simulink model "AVIC_model"  (R2015b)
settings: Solver=ode45  StartTime=0.0  StopTime=simtime  RelTol=1e-3
values from neighbouring files (symbols this model uses):
  A = 1    [simulation.m]
  a1 = 1    [simulation.m]
  a2 = 3    [simulation.m]
  a3 = 3    [simulation.m]
  Amp1 = Ampl/1000000    (= 134.217728)    [simulation.m]
  b1 = 1    [simulation.m]
  B2 = 8    [simulation.m]
  C = 32    [simulation.m]
  c1 = 1    [simulation.m]
  c2 = 1    [simulation.m]
  c3 = 1    [simulation.m]
  finrad = 2*pi/(N)*f0*clk    [simulation.m]
  FSC = 2^27    (= 134217728)    [simulation.m]
  SAT = 127    [simulation.m]
  Ts = 1/clk    (= 1.62760416667e-07)    [simulation.m]
libraries: simulink x298
(part 2 of 5)

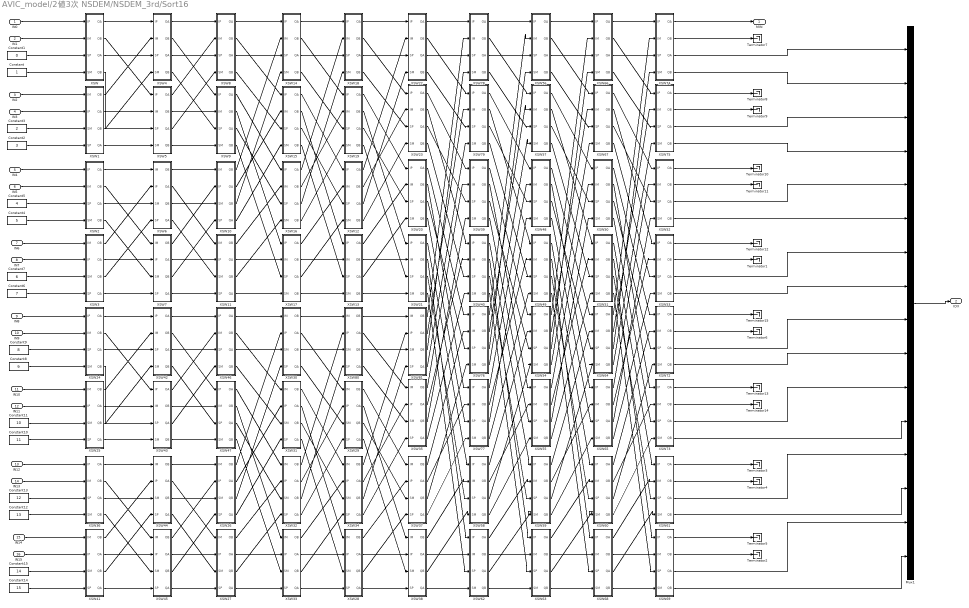
== system AVIC_model/2値3次 NSDEM/NSDEM_3rd/Sort16 ==
  IN0 : Inport
  IN1 : Inport  Port=2
  IN2 : Inport  Port=3
  IN3 : Inport  Port=4
  IN4 : Inport  Port=5
  IN5 : Inport  Port=6
  IN6 : Inport  Port=7
  IN7 : Inport  Port=8
  IN8 : Inport  Port=9
  IN9 : Inport  Port=10
  IN10 : Inport  Port=11
  IN11 : Inport  Port=12
  IN12 : Inport  Port=13
  IN13 : Inport  Port=14
  IN14 : Inport  Port=15
  IN15 : Inport  Port=16
  Constant : Constant
  Constant1 : Constant  Value=0
  Constant10 : Constant  Value=11
  Constant11 : Constant  Value=10
  Constant12 : Constant  Value=13
  Constant13 : Constant  Value=12
  Constant14 : Constant  Value=15
  Constant15 : Constant  Value=14
  Constant2 : Constant  Value=3
  Constant3 : Constant  Value=2
  Constant4 : Constant  Value=5
  Constant5 : Constant  Value=4
  Constant6 : Constant  Value=7
  Constant7 : Constant  Value=6
  Constant8 : Constant  Value=9
  Constant9 : Constant  Value=8
  Mux1 : Mux  Inputs=16
  Terminator{1..15} (15 alike) : Terminator
  XSW : Subsystem
  XSW1 : Subsystem
  XSW10 : Subsystem
  XSW11 : Subsystem
  XSW12 : Subsystem
  XSW13 : Subsystem
  XSW14 : Subsystem
  XSW15 : Subsystem
  XSW16 : Subsystem
  XSW17 : Subsystem
  XSW18 : Subsystem
  XSW19 : Subsystem
  XSW2 : Subsystem
  XSW20 : Subsystem
  XSW21 : Subsystem
  XSW22 : Subsystem
  XSW23 : Subsystem
  XSW24 : Subsystem
  XSW25 : Subsystem
  XSW26 : Subsystem
  XSW27 : Subsystem
  XSW28 : Subsystem
  XSW29 : Subsystem
  XSW3 : Subsystem
  XSW30 : Subsystem
  XSW31 : Subsystem
  XSW32 : Subsystem
  XSW33 : Subsystem
  XSW34 : Subsystem
  XSW35 : Subsystem
  XSW36 : Subsystem
  XSW37 : Subsystem
  XSW38 : Subsystem
  XSW39 : Subsystem
  XSW4 : Subsystem
  XSW40 : Subsystem
  XSW41 : Subsystem
  XSW42 : Subsystem
  XSW43 : Subsystem
  XSW44 : Subsystem
  XSW45 : Subsystem
  XSW46 : Subsystem
  XSW47 : Subsystem
  XSW48 : Subsystem
  XSW49 : Subsystem
  XSW5 : Subsystem
  XSW50 : Subsystem
  XSW51 : Subsystem
  XSW52 : Subsystem
  XSW53 : Subsystem
  XSW54 : Subsystem
  XSW55 : Subsystem
  XSW56 : Subsystem
  XSW57 : Subsystem
  XSW58 : Subsystem
  XSW59 : Subsystem
  XSW6 : Subsystem
  XSW60 : Subsystem
  XSW61 : Subsystem
  XSW62 : Subsystem
  XSW63 : Subsystem
  XSW64 : Subsystem
  XSW65 : Subsystem
  XSW66 : Subsystem
  XSW67 : Subsystem
  XSW68 : Subsystem
  XSW69 : Subsystem
  XSW7 : Subsystem
  XSW72 : Subsystem
  XSW73 : Subsystem
  XSW74 : Subsystem
  XSW75 : Subsystem
  XSW76 : Subsystem
  XSW77 : Subsystem
  XSW78 : Subsystem
  XSW79 : Subsystem
  XSW8 : Subsystem
  XSW80 : Subsystem
  XSW81 : Subsystem
  XSW9 : Subsystem
  MIN : Outport
  IDX : Outport  Port=2
  wires:
  XSW/1(OA) -> XSW4/1(IP)
  XSW/2(OB) -> XSW5/1(IP)
  XSW/3(QA) -> XSW4/3(SP)
  XSW/4(QB) -> XSW5/3(SP)
  XSW1/4(QA) -> XSW5/4(SM)
  XSW1/3(QB) -> XSW4/4(SM)
  XSW1/2(OA) -> XSW5/2(IM)
  XSW1/1(OB) -> XSW4/2(IM)
  XSW2/1(OA) -> XSW6/1(IM)
  XSW2/2(OB) -> XSW7/1(IM)
  XSW2/3(QA) -> XSW6/3(SM)
  XSW2/4(QB) -> XSW7/3(SM)
  XSW3/4(QA) -> XSW7/4(SP)
  XSW3/2(OA) -> XSW7/2(IP)
  XSW3/3(QB) -> XSW6/4(SP)
  XSW3/1(OB) -> XSW6/2(IP)
  XSW4/1(OA) -> XSW8/1(IP)
  XSW4/3(QA) -> XSW8/3(SP)
  XSW4/2(OB) -> XSW9/1(IP)
  XSW4/4(QB) -> XSW9/3(SP)
  XSW5/4(QB) -> XSW9/4(SM)
  XSW5/2(OB) -> XSW9/2(IM)
  XSW5/3(QA) -> XSW8/4(SM)
  XSW5/1(OA) -> XSW8/2(IM)
  XSW6/1(OB) -> XSW10/1(IM)
  XSW6/3(QB) -> XSW10/3(SM)
  XSW6/2(OA) -> XSW11/1(IM)
  XSW6/4(QA) -> XSW11/3(SM)
  XSW7/4(QA) -> XSW11/4(SP)
  XSW7/2(OA) -> XSW11/2(IP)
  XSW7/3(QB) -> XSW10/4(SP)
  XSW7/1(OB) -> XSW10/2(IP)
  XSW8/1(OA) -> XSW14/1(IP)
  XSW8/2(OB) -> XSW15/1(IP)
  XSW9/1(OA) -> XSW16/1(IP)
  XSW9/2(OB) -> XSW17/1(IP)
  XSW11/4(QA) -> XSW17/4(SM)
  XSW11/2(OA) -> XSW17/2(IM)
  XSW11/3(QB) -> XSW16/4(SM)
  XSW11/1(OB) -> XSW16/2(IM)
  XSW8/3(QA) -> XSW14/3(SP)
  XSW8/4(QB) -> XSW15/3(SP)
  XSW9/3(QA) -> XSW16/3(SP)
  XSW9/4(QB) -> XSW17/3(SP)
  XSW10/4(QA) -> XSW15/4(SM)
  XSW10/2(OA) -> XSW15/2(IM)
  XSW10/3(QB) -> XSW14/4(SM)
  XSW10/1(OB) -> XSW14/2(IM)
  XSW14/1(OA) -> XSW18/1(IP)
  XSW14/3(QA) -> XSW18/3(SP)
  XSW14/2(OB) -> XSW19/1(IP)
  XSW14/4(QB) -> XSW19/3(SP)
  XSW15/1(OA) -> XSW12/1(IP)
  XSW15/3(QA) -> XSW12/3(SP)
  XSW15/2(OB) -> XSW13/1(IP)
  XSW15/4(QB) -> XSW13/3(SP)
  XSW17/4(QB) -> XSW13/4(SM)
  XSW17/2(OB) -> XSW13/2(IM)
  XSW17/3(QA) -> XSW12/4(SM)
  XSW17/1(OA) -> XSW12/2(IM)
  XSW16/4(QB) -> XSW19/4(SM)
  XSW16/2(OB) -> XSW19/2(IM)
  XSW16/3(QA) -> XSW18/4(SM)
  XSW16/1(OA) -> XSW18/2(IM)
  XSW18/1(OA) -> XSW22/1(IP)
  XSW18/3(QA) -> XSW22/3(SP)
  XSW18/2(OB) -> XSW23/1(IP)
  XSW18/4(QB) -> XSW23/3(SP)
  XSW19/1(OA) -> XSW20/1(IP)
  XSW19/3(QA) -> XSW20/3(SP)
  XSW19/2(OB) -> XSW21/1(IP)
  XSW19/4(QB) -> XSW21/3(SP)
  XSW13/4(QB) -> XSW21/4(SM)
  XSW13/2(OB) -> XSW21/2(IM)
  XSW13/3(QA) -> XSW20/4(SM)
  XSW13/1(OA) -> XSW20/2(IM)
  XSW12/4(QB) -> XSW23/4(SM)
  XSW12/2(OB) -> XSW23/2(IM)
  XSW12/3(QA) -> XSW22/4(SM)
  XSW12/1(OA) -> XSW22/2(IM)
  XSW24/1(OA) -> XSW42/1(IP)
  XSW24/2(OB) -> XSW43/1(IP)
  XSW24/3(QA) -> XSW42/3(SP)
  XSW24/4(QB) -> XSW43/3(SP)
  XSW25/4(QA) -> XSW43/4(SM)
  XSW25/3(QB) -> XSW42/4(SM)
  XSW25/2(OA) -> XSW43/2(IM)
  XSW25/1(OB) -> XSW42/2(IM)
  XSW36/1(OA) -> XSW44/1(IM)
  XSW36/2(OB) -> XSW45/1(IM)
  XSW36/3(QA) -> XSW44/3(SM)
  XSW36/4(QB) -> XSW45/3(SM)
  XSW41/4(QA) -> XSW45/4(SP)
  XSW41/2(OA) -> XSW45/2(IP)
  XSW41/3(QB) -> XSW44/4(SP)
  XSW41/1(OB) -> XSW44/2(IP)
  XSW42/1(OA) -> XSW46/1(IP)
  XSW42/3(QA) -> XSW46/3(SP)
  XSW42/2(OB) -> XSW47/1(IP)
  XSW42/4(QB) -> XSW47/3(SP)
  XSW43/4(QB) -> XSW47/4(SM)
  XSW43/2(OB) -> XSW47/2(IM)
  XSW43/3(QA) -> XSW46/4(SM)
  XSW43/1(OA) -> XSW46/2(IM)
  XSW44/1(OB) -> XSW26/1(IM)
  XSW44/3(QB) -> XSW26/3(SM)
  XSW44/2(OA) -> XSW27/1(IM)
  XSW44/4(QA) -> XSW27/3(SM)
  XSW45/4(QA) -> XSW27/4(SP)
  XSW45/2(OA) -> XSW27/2(IP)
  XSW45/3(QB) -> XSW26/4(SP)
  XSW45/1(OB) -> XSW26/2(IP)
  XSW46/1(OA) -> XSW30/1(IM)
  XSW46/2(OB) -> XSW31/1(IM)
  XSW47/1(OA) -> XSW32/1(IM)
  XSW47/2(OB) -> XSW33/1(IM)
  XSW27/4(QA) -> XSW33/4(SP)
  XSW27/2(OA) -> XSW33/2(IP)
  XSW27/3(QB) -> XSW32/4(SP)
  XSW27/1(OB) -> XSW32/2(IP)
  XSW46/3(QA) -> XSW30/3(SM)
  XSW46/4(QB) -> XSW31/3(SM)
  XSW47/3(QA) -> XSW32/3(SM)
  XSW47/4(QB) -> XSW33/3(SM)
  XSW26/4(QA) -> XSW31/4(SP)
  XSW26/2(OA) -> XSW31/2(IP)
  XSW26/3(QB) -> XSW30/4(SP)
  XSW26/1(OB) -> XSW30/2(IP)
  XSW30/1(OB) -> XSW80/1(IM)
  XSW30/3(QB) -> XSW80/3(SM)
  XSW30/2(OA) -> XSW29/1(IM)
  XSW30/4(QA) -> XSW29/3(SM)
  XSW31/1(OB) -> XSW34/1(IM)
  XSW31/3(QB) -> XSW34/3(SM)
  XSW31/2(OA) -> XSW28/1(IM)
  XSW31/4(QA) -> XSW28/3(SM)
  XSW33/4(QA) -> XSW28/4(SP)
  XSW33/2(OA) -> XSW28/2(IP)
  XSW33/3(QB) -> XSW34/4(SP)
  XSW33/1(OB) -> XSW34/2(IP)
  XSW32/4(QA) -> XSW29/4(SP)
  XSW32/2(OA) -> XSW29/2(IP)
  XSW32/3(QB) -> XSW80/4(SP)
  XSW32/1(OB) -> XSW80/2(IP)
  XSW80/1(OB) -> XSW81/1(IM)
  XSW80/3(QB) -> XSW81/3(SM)
  XSW80/2(OA) -> XSW35/1(IM)
  XSW80/4(QA) -> XSW35/3(SM)
  XSW29/1(OB) -> XSW37/1(IM)
  XSW29/3(QB) -> XSW37/3(SM)
  XSW29/2(OA) -> XSW38/1(IM)
  XSW29/4(QA) -> XSW38/3(SM)
  XSW28/4(QA) -> XSW38/4(SP)
  XSW28/2(OA) -> XSW38/2(IP)
  XSW28/3(QB) -> XSW37/4(SP)
  XSW28/1(OB) -> XSW37/2(IP)
  XSW34/4(QA) -> XSW35/4(SP)
  XSW34/2(OA) -> XSW35/2(IP)
  XSW34/3(QB) -> XSW81/4(SP)
  XSW34/1(OB) -> XSW81/2(IP)
  XSW22/1(OA) -> XSW78/1(IP)
  XSW22/2(OB) -> XSW79/1(IP)
  XSW23/1(OA) -> XSW39/1(IP)
  XSW23/2(OB) -> XSW40/1(IP)
  XSW20/1(OA) -> XSW76/1(IP)
  XSW20/2(OB) -> XSW77/1(IP)
  XSW21/1(OA) -> XSW58/1(IP)
  XSW21/2(OB) -> XSW62/1(IP)
  XSW81/1(OB) -> XSW78/2(IM)
  XSW81/2(OA) -> XSW79/2(IM)
  XSW35/1(OB) -> XSW39/2(IM)
  XSW35/2(OA) -> XSW40/2(IM)
  XSW37/1(OB) -> XSW76/2(IM)
  XSW37/2(OA) -> XSW77/2(IM)
  XSW38/1(OB) -> XSW58/2(IM)
  XSW38/2(OA) -> XSW62/2(IM)
  XSW22/3(QA) -> XSW78/3(SP)
  XSW22/4(QB) -> XSW79/3(SP)
  XSW23/3(QA) -> XSW39/3(SP)
  XSW23/4(QB) -> XSW40/3(SP)
  XSW20/3(QA) -> XSW76/3(SP)
  XSW20/4(QB) -> XSW77/3(SP)
  XSW21/3(QA) -> XSW58/3(SP)
  XSW21/4(QB) -> XSW62/3(SP)
  XSW81/3(QB) -> XSW78/4(SM)
  XSW81/4(QA) -> XSW79/4(SM)
  XSW35/3(QB) -> XSW39/4(SM)
  XSW35/4(QA) -> XSW40/4(SM)
  XSW37/3(QB) -> XSW76/4(SM)
  XSW37/4(QA) -> XSW77/4(SM)
  XSW38/3(QB) -> XSW58/4(SM)
  XSW38/4(QA) -> XSW62/4(SM)
  XSW78/1(OA) -> XSW56/1(IP)
  XSW78/2(OB) -> XSW57/1(IP)
  XSW79/1(OA) -> XSW48/1(IP)
  XSW79/2(OB) -> XSW49/1(IP)
  XSW39/1(OA) -> XSW54/1(IP)
  XSW39/2(OB) -> XSW55/1(IP)
  XSW40/1(OA) -> XSW59/1(IP)
  XSW40/2(OB) -> XSW63/1(IP)
  XSW76/1(OA) -> XSW56/2(IM)
  XSW76/2(OB) -> XSW57/2(IM)
  XSW77/1(OA) -> XSW48/2(IM)
  XSW77/2(OB) -> XSW49/2(IM)
  XSW58/1(OA) -> XSW54/2(IM)
  XSW58/2(OB) -> XSW55/2(IM)
  XSW62/1(OA) -> XSW59/2(IM)
  XSW62/2(OB) -> XSW63/2(IM)
  XSW78/3(QA) -> XSW56/3(SP)
  XSW78/4(QB) -> XSW57/3(SP)
  XSW79/3(QA) -> XSW48/3(SP)
  XSW79/4(QB) -> XSW49/3(SP)
  XSW39/3(QA) -> XSW54/3(SP)
  XSW39/4(QB) -> XSW55/3(SP)
  XSW40/3(QA) -> XSW59/3(SP)
  XSW40/4(QB) -> XSW63/3(SP)
  XSW76/3(QA) -> XSW56/4(SM)
  XSW76/4(QB) -> XSW57/4(SM)
  XSW77/3(QA) -> XSW48/4(SM)
  XSW77/4(QB) -> XSW49/4(SM)
  XSW58/3(QA) -> XSW54/4(SM)
  XSW58/4(QB) -> XSW55/4(SM)
  XSW62/3(QA) -> XSW59/4(SM)
  XSW62/4(QB) -> XSW63/4(SM)
  XSW56/1(OA) -> XSW66/1(IP)
  XSW56/2(OB) -> XSW67/1(IP)
  XSW57/1(OA) -> XSW50/1(IP)
  XSW57/2(OB) -> XSW51/1(IP)
  XSW48/1(OA) -> XSW64/1(IP)
  XSW48/2(OB) -> XSW65/1(IP)
  XSW49/1(OA) -> XSW60/1(IP)
  XSW49/2(OB) -> XSW68/1(IP)
  XSW54/1(OA) -> XSW66/2(IM)
  XSW54/2(OB) -> XSW67/2(IM)
  XSW55/1(OA) -> XSW50/2(IM)
  XSW55/2(OB) -> XSW51/2(IM)
  XSW59/1(OA) -> XSW64/2(IM)
  XSW59/2(OB) -> XSW65/2(IM)
  XSW63/1(OA) -> XSW60/2(IM)
  XSW63/2(OB) -> XSW68/2(IM)
  XSW56/3(QA) -> XSW66/3(SP)
  XSW56/4(QB) -> XSW67/3(SP)
  XSW57/3(QA) -> XSW50/3(SP)
  XSW57/4(QB) -> XSW51/3(SP)
  XSW48/3(QA) -> XSW64/3(SP)
  XSW48/4(QB) -> XSW65/3(SP)
  XSW49/3(QA) -> XSW60/3(SP)
  XSW49/4(QB) -> XSW68/3(SP)
  XSW54/3(QA) -> XSW66/4(SM)
  XSW54/4(QB) -> XSW67/4(SM)
  XSW55/3(QA) -> XSW50/4(SM)
  XSW55/4(QB) -> XSW51/4(SM)
  XSW59/3(QA) -> XSW64/4(SM)
  XSW59/4(QB) -> XSW65/4(SM)
  XSW63/3(QA) -> XSW60/4(SM)
  XSW63/4(QB) -> XSW68/4(SM)
  XSW66/1(OA) -> XSW74/1(IP)
  XSW66/2(OB) -> XSW75/1(IP)
  XSW67/1(OA) -> XSW52/1(IP)
  XSW67/2(OB) -> XSW53/1(IP)
  XSW50/1(OA) -> XSW72/1(IP)
  XSW50/2(OB) -> XSW73/1(IP)
  XSW51/1(OA) -> XSW61/1(IP)
  XSW51/2(OB) -> XSW69/1(IP)
  XSW64/1(OA) -> XSW74/2(IM)
  XSW64/2(OB) -> XSW75/2(IM)
  XSW65/1(OA) -> XSW52/2(IM)
  XSW65/2(OB) -> XSW53/2(IM)
  XSW60/1(OA) -> XSW72/2(IM)
  XSW60/2(OB) -> XSW73/2(IM)
  XSW68/1(OA) -> XSW61/2(IM)
  XSW68/2(OB) -> XSW69/2(IM)
  XSW66/3(QA) -> XSW74/3(SP)
  XSW66/4(QB) -> XSW75/3(SP)
  XSW67/3(QA) -> XSW52/3(SP)
  XSW67/4(QB) -> XSW53/3(SP)
  XSW50/3(QA) -> XSW72/3(SP)
  XSW50/4(QB) -> XSW73/3(SP)
  XSW51/3(QA) -> XSW61/3(SP)
  XSW51/4(QB) -> XSW69/3(SP)
  XSW64/3(QA) -> XSW74/4(SM)
  XSW64/4(QB) -> XSW75/4(SM)
  XSW65/3(QA) -> XSW52/4(SM)
  XSW65/4(QB) -> XSW53/4(SM)
  XSW60/3(QA) -> XSW72/4(SM)
  XSW60/4(QB) -> XSW73/4(SM)
  XSW68/3(QA) -> XSW61/4(SM)
  XSW68/4(QB) -> XSW69/4(SM)
  XSW74/1(OA) -> MIN/1
  XSW74/2(OB) -> Terminator7/1
  XSW75/1(OA) -> Terminator8/1
  XSW75/2(OB) -> Terminator9/1
  XSW52/1(OA) -> Terminator10/1
  XSW52/2(OB) -> Terminator11/1
  XSW53/1(OA) -> Terminator12/1
  XSW53/2(OB) -> Terminator1/1
  XSW72/1(OA) -> Terminator15/1
  XSW72/2(OB) -> Terminator6/1
  XSW73/1(OA) -> Terminator13/1
  XSW73/2(OB) -> Terminator14/1
  XSW61/1(OA) -> Terminator3/1
  XSW61/2(OB) -> Terminator4/1
  XSW69/1(OA) -> Terminator5/1
  XSW69/2(OB) -> Terminator2/1
  IN0/1 -> XSW/1(IP)
  IN1/1 -> XSW/2(IM)
  Constant1/1 -> XSW/3(SP)
  Constant/1 -> XSW/4(SM)
  IN2/1 -> XSW1/1(IM)
  IN3/1 -> XSW1/2(IP)
  Constant3/1 -> XSW1/3(SM)
  Constant2/1 -> XSW1/4(SP)
  IN4/1 -> XSW2/1(IP)
  IN5/1 -> XSW2/2(IM)
  Constant5/1 -> XSW2/3(SP)
  Constant4/1 -> XSW2/4(SM)
  IN6/1 -> XSW3/1(IM)
  IN7/1 -> XSW3/2(IP)
  Constant7/1 -> XSW3/3(SM)
  Constant6/1 -> XSW3/4(SP)
  IN8/1 -> XSW24/1(IP)
  IN9/1 -> XSW24/2(IM)
  Constant9/1 -> XSW24/3(SP)
  Constant8/1 -> XSW24/4(SM)
  IN10/1 -> XSW25/1(IM)
  IN11/1 -> XSW25/2(IP)
  Constant11/1 -> XSW25/3(SM)
  Constant10/1 -> XSW25/4(SP)
  IN12/1 -> XSW36/1(IP)
  IN13/1 -> XSW36/2(IM)
  Constant13/1 -> XSW36/3(SP)
  Constant12/1 -> XSW36/4(SM)
  IN14/1 -> XSW41/1(IM)
  IN15/1 -> XSW41/2(IP)
  Constant15/1 -> XSW41/3(SM)
  Constant14/1 -> XSW41/4(SP)
  XSW53/4(QB) -> Mux1/8
  XSW74/3(QA) -> Mux1/1
  XSW74/4(QB) -> Mux1/2
  XSW75/3(QA) -> Mux1/3
  XSW75/4(QB) -> Mux1/4
  XSW52/3(QA) -> Mux1/5
  XSW52/4(QB) -> Mux1/6
  XSW53/3(QA) -> Mux1/7
  XSW72/3(QA) -> Mux1/9
  XSW72/4(QB) -> Mux1/10
  XSW73/3(QA) -> Mux1/11
  XSW73/4(QB) -> Mux1/12
  XSW61/3(QA) -> Mux1/13
  XSW61/4(QB) -> Mux1/14
  XSW69/3(QA) -> Mux1/15
  XSW69/4(QB) -> Mux1/16
  Mux1/1 -> IDX/1

== system AVIC_model/ESB/Subsystem4/Subsystem ==
  In1 : Inport
  Combinatorial Logic{,2,4..5} (4 alike) : CombinatorialLogic  TruthTable=[0 0 0 0 0 0 0 0;0 0 0 0 0 0 0 0]
  Combinatorial Logic1 : CombinatorialLogic  TruthTable=[0 0 0 0 0 0 0 0;0 0 0 0 0 0 0 1]
  Combinatorial Logic3 : CombinatorialLogic  TruthTable=[0 0 0 0 0 0 0 0;0 0 0 0 0 0 0 1]
  Compare To Constnt : simulink/Logic and Bit Operations/Compare To Constant  relop===  const=0  OutDataTypeStr=boolean  ZeroCross=off
  Compare To Constnt1 : simulink/Logic and Bit Operations/Compare To Constant  relop===  const=1  OutDataTypeStr=boolean  ZeroCross=off
  Compare To Constnt2 : simulink/Logic and Bit Operations/Compare To Constant  relop===  const=2  OutDataTypeStr=boolean  ZeroCross=off
  Logical Operator : Logic  Operator=OR  Inputs=3  AllPortsSameDT=off  OutDataTypeStr=boolean
  Logical Operator1 : Logic  Operator=OR  Inputs=3  AllPortsSameDT=off  OutDataTypeStr=boolean
  "P1 " : Outport
  "N1 " : Outport  Port=2
  wires:
  Logical Operator/1 -> "P1 "/1
  In1/1 -> Compare To Constnt/1, Compare To Constnt1/1, Compare To Constnt2/1
  Combinatorial Logic/1 -> Logical Operator/1
  Combinatorial Logic2/1 -> Logical Operator/2
  Combinatorial Logic1/1 -> Logical Operator/3
  Logical Operator1/1 -> "N1 "/1
  Compare To Constnt/1 -> Combinatorial Logic3/1, Combinatorial Logic/1
  Compare To Constnt1/1 -> Combinatorial Logic4/1, Combinatorial Logic2/1
  Compare To Constnt2/1 -> Combinatorial Logic5/1, Combinatorial Logic1/1
  Combinatorial Logic3/1 -> Logical Operator1/1
  Combinatorial Logic4/1 -> Logical Operator1/2
  Combinatorial Logic5/1 -> Logical Operator1/3

== system AVIC_model/ESB/Subsystem4/Subsystem1 ==
  In1 : Inport
  Combinatorial Logic{,2,4..5} (4 alike) : CombinatorialLogic  TruthTable=[0 0 0 0 0 0 0 0;0 0 0 0 0 0 0 0]
  Combinatorial Logic1 : CombinatorialLogic  TruthTable=[0 0 0 0 0 0 0 0;0 0 0 0 0 0 1 0]
  Combinatorial Logic3 : CombinatorialLogic  TruthTable=[0 0 0 0 0 0 0 0;0 0 0 0 0 0 1 0]
  Compare To Constnt : simulink/Logic and Bit Operations/Compare To Constant  relop===  const=0  OutDataTypeStr=boolean  ZeroCross=off
  Compare To Constnt1 : simulink/Logic and Bit Operations/Compare To Constant  relop===  const=1  OutDataTypeStr=boolean  ZeroCross=off
  Compare To Constnt2 : simulink/Logic and Bit Operations/Compare To Constant  relop===  const=2  OutDataTypeStr=boolean  ZeroCross=off
  Logical Operator : Logic  Operator=OR  Inputs=3  AllPortsSameDT=off  OutDataTypeStr=boolean
  Logical Operator1 : Logic  Operator=OR  Inputs=3  AllPortsSameDT=off  OutDataTypeStr=boolean
  "P1 " : Outport
  "N1 " : Outport  Port=2
  wires:
  Logical Operator/1 -> "P1 "/1
  In1/1 -> Compare To Constnt/1, Compare To Constnt1/1, Compare To Constnt2/1
  Combinatorial Logic/1 -> Logical Operator/1
  Combinatorial Logic2/1 -> Logical Operator/2
  Combinatorial Logic1/1 -> Logical Operator/3
  Logical Operator1/1 -> "N1 "/1
  Compare To Constnt/1 -> Combinatorial Logic3/1, Combinatorial Logic/1
  Compare To Constnt1/1 -> Combinatorial Logic4/1, Combinatorial Logic2/1
  Compare To Constnt2/1 -> Combinatorial Logic5/1, Combinatorial Logic1/1
  Combinatorial Logic3/1 -> Logical Operator1/1
  Combinatorial Logic4/1 -> Logical Operator1/2
  Combinatorial Logic5/1 -> Logical Operator1/3

== system AVIC_model/ESB/Subsystem4/Subsystem2 ==
  In1 : Inport
  Combinatorial Logic{,2,4..5} (4 alike) : CombinatorialLogic  TruthTable=[0 0 0 0 0 0 0 0;0 0 0 0 0 0 0 0]
  Combinatorial Logic1 : CombinatorialLogic  TruthTable=[0 0 0 0 0 0 0 0;0 0 0 0 0 1 0 0]
  Combinatorial Logic3 : CombinatorialLogic  TruthTable=[0 0 0 0 0 0 0 0;0 0 0 0 0 1 0 0]
  Compare To Constnt : simulink/Logic and Bit Operations/Compare To Constant  relop===  const=0  OutDataTypeStr=boolean  ZeroCross=off
  Compare To Constnt1 : simulink/Logic and Bit Operations/Compare To Constant  relop===  const=1  OutDataTypeStr=boolean  ZeroCross=off
  Compare To Constnt2 : simulink/Logic and Bit Operations/Compare To Constant  relop===  const=2  OutDataTypeStr=boolean  ZeroCross=off
  Logical Operator : Logic  Operator=OR  Inputs=3  AllPortsSameDT=off  OutDataTypeStr=boolean
  Logical Operator1 : Logic  Operator=OR  Inputs=3  AllPortsSameDT=off  OutDataTypeStr=boolean
  "P1 " : Outport
  "N1 " : Outport  Port=2
  wires:
  Logical Operator/1 -> "P1 "/1
  In1/1 -> Compare To Constnt/1, Compare To Constnt1/1, Compare To Constnt2/1
  Combinatorial Logic/1 -> Logical Operator/1
  Combinatorial Logic2/1 -> Logical Operator/2
  Combinatorial Logic1/1 -> Logical Operator/3
  Logical Operator1/1 -> "N1 "/1
  Compare To Constnt/1 -> Combinatorial Logic3/1, Combinatorial Logic/1
  Compare To Constnt1/1 -> Combinatorial Logic4/1, Combinatorial Logic2/1
  Compare To Constnt2/1 -> Combinatorial Logic5/1, Combinatorial Logic1/1
  Combinatorial Logic3/1 -> Logical Operator1/1
  Combinatorial Logic4/1 -> Logical Operator1/2
  Combinatorial Logic5/1 -> Logical Operator1/3

== system AVIC_model/ESB/Subsystem4/Subsystem3 ==
  In1 : Inport
  Combinatorial Logic{,2,4..5} (4 alike) : CombinatorialLogic  TruthTable=[0 0 0 0 0 0 0 0;0 0 0 0 0 0 0 0]
  Combinatorial Logic1 : CombinatorialLogic  TruthTable=[0 0 0 0 0 0 0 0;0 0 0 0 1 0 0 0]
  Combinatorial Logic3 : CombinatorialLogic  TruthTable=[0 0 0 0 0 0 0 0;0 0 0 0 1 0 0 0]
  Compare To Constnt : simulink/Logic and Bit Operations/Compare To Constant  relop===  const=0  OutDataTypeStr=boolean  ZeroCross=off
  Compare To Constnt1 : simulink/Logic and Bit Operations/Compare To Constant  relop===  const=1  OutDataTypeStr=boolean  ZeroCross=off
  Compare To Constnt2 : simulink/Logic and Bit Operations/Compare To Constant  relop===  const=2  OutDataTypeStr=boolean  ZeroCross=off
  Logical Operator : Logic  Operator=OR  Inputs=3  AllPortsSameDT=off  OutDataTypeStr=boolean
  Logical Operator1 : Logic  Operator=OR  Inputs=3  AllPortsSameDT=off  OutDataTypeStr=boolean
  "P1 " : Outport
  "N1 " : Outport  Port=2
  wires:
  Logical Operator/1 -> "P1 "/1
  In1/1 -> Compare To Constnt/1, Compare To Constnt1/1, Compare To Constnt2/1
  Combinatorial Logic/1 -> Logical Operator/1
  Combinatorial Logic2/1 -> Logical Operator/2
  Combinatorial Logic1/1 -> Logical Operator/3
  Logical Operator1/1 -> "N1 "/1
  Compare To Constnt/1 -> Combinatorial Logic3/1, Combinatorial Logic/1
  Compare To Constnt1/1 -> Combinatorial Logic4/1, Combinatorial Logic2/1
  Compare To Constnt2/1 -> Combinatorial Logic5/1, Combinatorial Logic1/1
  Combinatorial Logic3/1 -> Logical Operator1/1
  Combinatorial Logic4/1 -> Logical Operator1/2
  Combinatorial Logic5/1 -> Logical Operator1/3

== system AVIC_model/ESB/Subsystem4/Subsystem4 ==
  In1 : Inport
  Combinatorial Logic{,2,4..5} (4 alike) : CombinatorialLogic  TruthTable=[0 0 0 0 0 0 0 0;0 0 0 0 0 0 0 0]
  Combinatorial Logic1 : CombinatorialLogic  TruthTable=[0 0 0 0 0 0 0 0;0 0 0 1 0 0 0 0]
  Combinatorial Logic3 : CombinatorialLogic  TruthTable=[0 0 0 0 0 0 0 0;0 0 0 1 0 0 0 0]
  Compare To Constnt : simulink/Logic and Bit Operations/Compare To Constant  relop===  const=0  OutDataTypeStr=boolean  ZeroCross=off
  Compare To Constnt1 : simulink/Logic and Bit Operations/Compare To Constant  relop===  const=1  OutDataTypeStr=boolean  ZeroCross=off
  Compare To Constnt2 : simulink/Logic and Bit Operations/Compare To Constant  relop===  const=2  OutDataTypeStr=boolean  ZeroCross=off
  Logical Operator : Logic  Operator=OR  Inputs=3  AllPortsSameDT=off  OutDataTypeStr=boolean
  Logical Operator1 : Logic  Operator=OR  Inputs=3  AllPortsSameDT=off  OutDataTypeStr=boolean
  "P1 " : Outport
  "N1 " : Outport  Port=2
  wires:
  Logical Operator/1 -> "P1 "/1
  In1/1 -> Compare To Constnt/1, Compare To Constnt1/1, Compare To Constnt2/1
  Combinatorial Logic/1 -> Logical Operator/1
  Combinatorial Logic2/1 -> Logical Operator/2
  Combinatorial Logic1/1 -> Logical Operator/3
  Logical Operator1/1 -> "N1 "/1
  Compare To Constnt/1 -> Combinatorial Logic3/1, Combinatorial Logic/1
  Compare To Constnt1/1 -> Combinatorial Logic4/1, Combinatorial Logic2/1
  Compare To Constnt2/1 -> Combinatorial Logic5/1, Combinatorial Logic1/1
  Combinatorial Logic3/1 -> Logical Operator1/1
  Combinatorial Logic4/1 -> Logical Operator1/2
  Combinatorial Logic5/1 -> Logical Operator1/3

== system AVIC_model/ESB/Subsystem4/Subsystem5 ==
  In1 : Inport
  Combinatorial Logic{,2,4..5} (4 alike) : CombinatorialLogic  TruthTable=[0 0 0 0 0 0 0 0;0 0 0 0 0 0 0 0]
  Combinatorial Logic1 : CombinatorialLogic  TruthTable=[0 0 0 0 0 0 0 0;0 0 1 0 0 0 0 0]
  Combinatorial Logic3 : CombinatorialLogic  TruthTable=[0 0 0 0 0 0 0 0;0 0 1 0 0 0 0 0]
  Compare To Constnt : simulink/Logic and Bit Operations/Compare To Constant  relop===  const=0  OutDataTypeStr=boolean  ZeroCross=off
  Compare To Constnt1 : simulink/Logic and Bit Operations/Compare To Constant  relop===  const=1  OutDataTypeStr=boolean  ZeroCross=off
  Compare To Constnt2 : simulink/Logic and Bit Operations/Compare To Constant  relop===  const=2  OutDataTypeStr=boolean  ZeroCross=off
  Logical Operator : Logic  Operator=OR  Inputs=3  AllPortsSameDT=off  OutDataTypeStr=boolean
  Logical Operator1 : Logic  Operator=OR  Inputs=3  AllPortsSameDT=off  OutDataTypeStr=boolean
  "P1 " : Outport
  "N1 " : Outport  Port=2
  wires:
  Logical Operator/1 -> "P1 "/1
  In1/1 -> Compare To Constnt/1, Compare To Constnt1/1, Compare To Constnt2/1
  Combinatorial Logic/1 -> Logical Operator/1
  Combinatorial Logic2/1 -> Logical Operator/2
  Combinatorial Logic1/1 -> Logical Operator/3
  Logical Operator1/1 -> "N1 "/1
  Compare To Constnt/1 -> Combinatorial Logic3/1, Combinatorial Logic/1
  Compare To Constnt1/1 -> Combinatorial Logic4/1, Combinatorial Logic2/1
  Compare To Constnt2/1 -> Combinatorial Logic5/1, Combinatorial Logic1/1
  Combinatorial Logic3/1 -> Logical Operator1/1
  Combinatorial Logic4/1 -> Logical Operator1/2
  Combinatorial Logic5/1 -> Logical Operator1/3

== system AVIC_model/ESB/Subsystem4/Subsystem6 ==
  In1 : Inport
  Combinatorial Logic{,2,4..5} (4 alike) : CombinatorialLogic  TruthTable=[0 0 0 0 0 0 0 0;0 0 0 0 0 0 0 0]
  Combinatorial Logic1 : CombinatorialLogic  TruthTable=[0 0 0 0 0 0 0 0;0 1 0 0 0 0 0 0]
  Combinatorial Logic3 : CombinatorialLogic  TruthTable=[0 0 0 0 0 0 0 0;0 1 0 0 0 0 0 0]
  Compare To Constnt : simulink/Logic and Bit Operations/Compare To Constant  relop===  const=0  OutDataTypeStr=boolean  ZeroCross=off
  Compare To Constnt1 : simulink/Logic and Bit Operations/Compare To Constant  relop===  const=1  OutDataTypeStr=boolean  ZeroCross=off
  Compare To Constnt2 : simulink/Logic and Bit Operations/Compare To Constant  relop===  const=2  OutDataTypeStr=boolean  ZeroCross=off
  Logical Operator : Logic  Operator=OR  Inputs=3  AllPortsSameDT=off  OutDataTypeStr=boolean
  Logical Operator1 : Logic  Operator=OR  Inputs=3  AllPortsSameDT=off  OutDataTypeStr=boolean
  "P1 " : Outport
  "N1 " : Outport  Port=2
  wires:
  Logical Operator/1 -> "P1 "/1
  In1/1 -> Compare To Constnt/1, Compare To Constnt1/1, Compare To Constnt2/1
  Combinatorial Logic/1 -> Logical Operator/1
  Combinatorial Logic2/1 -> Logical Operator/2
  Combinatorial Logic1/1 -> Logical Operator/3
  Logical Operator1/1 -> "N1 "/1
  Compare To Constnt/1 -> Combinatorial Logic3/1, Combinatorial Logic/1
  Compare To Constnt1/1 -> Combinatorial Logic4/1, Combinatorial Logic2/1
  Compare To Constnt2/1 -> Combinatorial Logic5/1, Combinatorial Logic1/1
  Combinatorial Logic3/1 -> Logical Operator1/1
  Combinatorial Logic4/1 -> Logical Operator1/2
  Combinatorial Logic5/1 -> Logical Operator1/3

== system AVIC_model/ESB/Subsystem4/Subsystem7 ==
  In1 : Inport
  Combinatorial Logic{,2,4..5} (4 alike) : CombinatorialLogic  TruthTable=[0 0 0 0 0 0 0 0;0 0 0 0 0 0 0 0]
  Combinatorial Logic1 : CombinatorialLogic  TruthTable=[0 0 0 0 0 0 0 0;1 0 0 0 0 0 0 0]
  Combinatorial Logic3 : CombinatorialLogic  TruthTable=[0 0 0 0 0 0 0 0;1 0 0 0 0 0 0 0]
  Compare To Constnt : simulink/Logic and Bit Operations/Compare To Constant  relop===  const=0  OutDataTypeStr=boolean  ZeroCross=off
  Compare To Constnt1 : simulink/Logic and Bit Operations/Compare To Constant  relop===  const=1  OutDataTypeStr=boolean  ZeroCross=off
  Compare To Constnt2 : simulink/Logic and Bit Operations/Compare To Constant  relop===  const=2  OutDataTypeStr=boolean  ZeroCross=off
  Logical Operator : Logic  Operator=OR  Inputs=3  AllPortsSameDT=off  OutDataTypeStr=boolean
  Logical Operator1 : Logic  Operator=OR  Inputs=3  AllPortsSameDT=off  OutDataTypeStr=boolean
  "P1 " : Outport
  "N1 " : Outport  Port=2
  wires:
  Logical Operator/1 -> "P1 "/1
  In1/1 -> Compare To Constnt/1, Compare To Constnt1/1, Compare To Constnt2/1
  Combinatorial Logic/1 -> Logical Operator/1
  Combinatorial Logic2/1 -> Logical Operator/2
  Combinatorial Logic1/1 -> Logical Operator/3
  Logical Operator1/1 -> "N1 "/1
  Compare To Constnt/1 -> Combinatorial Logic3/1, Combinatorial Logic/1
  Compare To Constnt1/1 -> Combinatorial Logic4/1, Combinatorial Logic2/1
  Compare To Constnt2/1 -> Combinatorial Logic5/1, Combinatorial Logic1/1
  Combinatorial Logic3/1 -> Logical Operator1/1
  Combinatorial Logic4/1 -> Logical Operator1/2
  Combinatorial Logic5/1 -> Logical Operator1/3

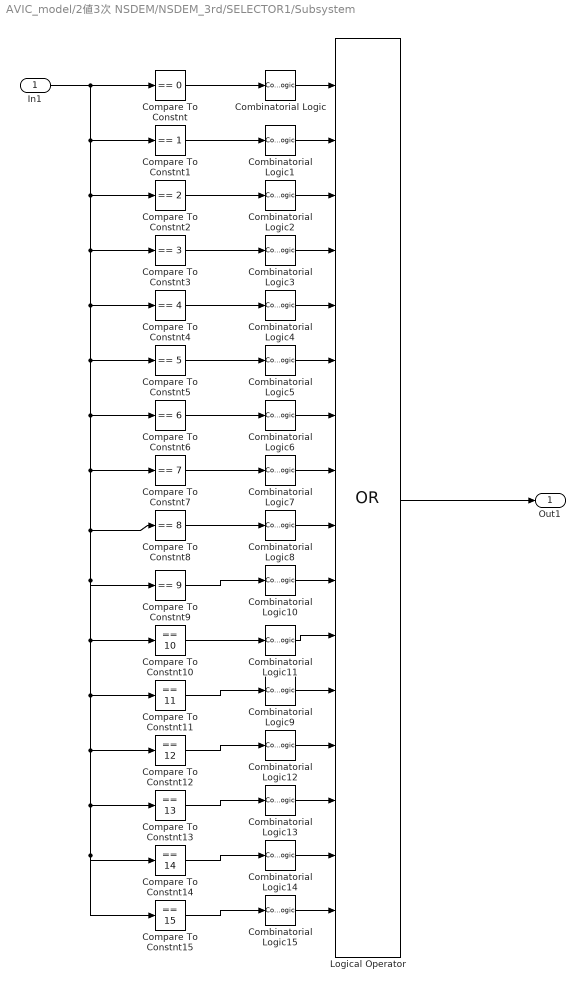
== system AVIC_model/2値3次 NSDEM/NSDEM_3rd/SELECTOR1/Subsystem ==
  In1 : Inport
  Combinatorial Logic : CombinatorialLogic  TruthTable=[0 0 0 0 0 0 0 0 0 0 0 0 0 0 0 0;1 0 0 0 0 0 0 0 0 0 0 0 0 0 0 0]
  Combinatorial Logic1 : CombinatorialLogic  TruthTable=[0 0 0 0 0 0 0 0 0 0 0 0 0 0 0 0; 0 1 0 0 0 0 0 0 0 0 0 0 0 0 0 0]
  Combinatorial Logic10 : CombinatorialLogic  TruthTable=[0 0 0 0 0 0 0 0 0 0 0 0 0 0 0 0;0 0 0 0 0 0 0 0 0 1 0 0 0 0 0 0]
  Combinatorial Logic11 : CombinatorialLogic  TruthTable=[0 0 0 0 0 0 0 0 0 0 0 0 0 0 0 0;0 0 0 0 0 0 0 0 0 0 1 0 0 0 0 0 ]
  Combinatorial Logic12 : CombinatorialLogic  TruthTable=[0 0 0 0 0 0 0 0 0 0 0 0 0 0 0 0;0 0 0 0 0 0 0 0 0 0 0 0 1 0 0 0]
  Combinatorial Logic13 : CombinatorialLogic  TruthTable=[0 0 0 0 0 0 0 0 0 0 0 0 0 0 0 0;0 0 0 0 0 0 0 0 0 0 0 0 0 1 0 0]
  Combinatorial Logic14 : CombinatorialLogic  TruthTable=[0 0 0 0 0 0 0 0 0 0 0 0 0 0 0 0;0 0 0 0 0 0 0 0 0 0 0 0 0 0 1 0]
  Combinatorial Logic15 : CombinatorialLogic  TruthTable=[0 0 0 0 0 0 0 0 0 0 0 0 0 0 0 0;0 0 0 0 0 0 0 0 0 0 0 0 0 0 0 1]
  Combinatorial Logic2 : CombinatorialLogic  TruthTable=[0 0 0 0 0 0 0 0 0 0 0 0 0 0 0 0;0 0 1 0 0 0 0 0 0 0 0 0 0 0 0 0]
  Combinatorial Logic3 : CombinatorialLogic  TruthTable=[0 0 0 0 0 0 0 0 0 0 0 0 0 0 0 0;0 0 0 1 0 0 0 0 0 0 0 0 0 0 0 0]
  Combinatorial Logic4 : CombinatorialLogic  TruthTable=[0 0 0 0 0 0 0 0 0 0 0 0 0 0 0 0;0 0 0 0 1 0 0 0 0 0 0 0 0 0 0 0]
  Combinatorial Logic5 : CombinatorialLogic  TruthTable=[0 0 0 0 0 0 0 0 0 0 0 0 0 0 0 0;0 0 0 0 0 1 0 0 0 0 0 0 0 0 0 0]
  Combinatorial Logic6 : CombinatorialLogic  TruthTable=[0 0 0 0 0 0 0 0 0 0 0 0 0 0 0 0;0 0 0 0 0 0 1 0 0 0 0 0 0 0 0 0]
  Combinatorial Logic7 : CombinatorialLogic  TruthTable=[0 0 0 0 0 0 0 0 0 0 0 0 0 0 0 0;0 0 0 0 0 0 0 1 0 0 0 0 0 0 0 0]
  Combinatorial Logic8 : CombinatorialLogic  TruthTable=[0 0 0 0 0 0 0 0 0 0 0 0 0 0 0 0;0 0 0 0 0 0 0 0 1 0 0 0 0 0 0 0]
  Combinatorial Logic9 : CombinatorialLogic  TruthTable=[0 0 0 0 0 0 0 0 0 0 0 0 0 0 0 0;0 0 0 0 0 0 0 0 0 0 0 1 0 0 0 0 ]
  Compare To Constnt : simulink/Logic and Bit Operations/Compare To Constant  relop===  const=0  OutDataTypeStr=boolean  ZeroCross=off
  Compare To Constnt1 : simulink/Logic and Bit Operations/Compare To Constant  relop===  const=1  OutDataTypeStr=boolean  ZeroCross=off
  Compare To Constnt10 : simulink/Logic and Bit Operations/Compare To Constant  relop===  const=10  OutDataTypeStr=boolean  ZeroCross=off
  Compare To Constnt11 : simulink/Logic and Bit Operations/Compare To Constant  relop===  const=11  OutDataTypeStr=boolean  ZeroCross=off
  Compare To Constnt12 : simulink/Logic and Bit Operations/Compare To Constant  relop===  const=12  OutDataTypeStr=boolean  ZeroCross=off
  Compare To Constnt13 : simulink/Logic and Bit Operations/Compare To Constant  relop===  const=13  OutDataTypeStr=boolean  ZeroCross=off
  Compare To Constnt14 : simulink/Logic and Bit Operations/Compare To Constant  relop===  const=14  OutDataTypeStr=boolean  ZeroCross=off
  Compare To Constnt15 : simulink/Logic and Bit Operations/Compare To Constant  relop===  const=15  OutDataTypeStr=boolean  ZeroCross=off
  Compare To Constnt2 : simulink/Logic and Bit Operations/Compare To Constant  relop===  const=2  OutDataTypeStr=boolean  ZeroCross=off
  Compare To Constnt3 : simulink/Logic and Bit Operations/Compare To Constant  relop===  const=3  OutDataTypeStr=boolean  ZeroCross=off
  Compare To Constnt4 : simulink/Logic and Bit Operations/Compare To Constant  relop===  const=4  OutDataTypeStr=boolean  ZeroCross=off
  Compare To Constnt5 : simulink/Logic and Bit Operations/Compare To Constant  relop===  const=5  OutDataTypeStr=boolean  ZeroCross=off
  Compare To Constnt6 : simulink/Logic and Bit Operations/Compare To Constant  relop===  const=6  OutDataTypeStr=boolean  ZeroCross=off
  Compare To Constnt7 : simulink/Logic and Bit Operations/Compare To Constant  relop===  const=7  OutDataTypeStr=boolean  ZeroCross=off
  Compare To Constnt8 : simulink/Logic and Bit Operations/Compare To Constant  relop===  const=8  OutDataTypeStr=boolean  ZeroCross=off
  Compare To Constnt9 : simulink/Logic and Bit Operations/Compare To Constant  relop===  const=9  OutDataTypeStr=boolean  ZeroCross=off
  Logical Operator : Logic  Operator=OR  Inputs=16  AllPortsSameDT=off  OutDataTypeStr=boolean
  Out1 : Outport
  wires:
  Logical Operator/1 -> Out1/1
  In1/1 -> Compare To Constnt/1, Compare To Constnt1/1, Compare To Constnt2/1, Compare To Constnt3/1, Compare To Constnt4/1, Compare To Constnt5/1, Compare To Constnt6/1, Compare To Constnt7/1, Compare To Constnt8/1, Compare To Constnt9/1, Compare To Constnt10/1, Compare To Constnt11/1, Compare To Constnt12/1, Compare To Constnt13/1, Compare To Constnt15/1, Compare To Constnt14/1
  Compare To Constnt/1 -> Combinatorial Logic/1
  Compare To Constnt1/1 -> Combinatorial Logic1/1
  Compare To Constnt2/1 -> Combinatorial Logic2/1
  Compare To Constnt3/1 -> Combinatorial Logic3/1
  Compare To Constnt4/1 -> Combinatorial Logic4/1
  Compare To Constnt5/1 -> Combinatorial Logic5/1
  Compare To Constnt6/1 -> Combinatorial Logic6/1
  Compare To Constnt7/1 -> Combinatorial Logic7/1
  Combinatorial Logic/1 -> Logical Operator/1
  Combinatorial Logic1/1 -> Logical Operator/2
  Combinatorial Logic2/1 -> Logical Operator/3
  Combinatorial Logic3/1 -> Logical Operator/4
  Combinatorial Logic4/1 -> Logical Operator/5
  Combinatorial Logic5/1 -> Logical Operator/6
  Combinatorial Logic6/1 -> Logical Operator/7
  Combinatorial Logic7/1 -> Logical Operator/8
  Compare To Constnt8/1 -> Combinatorial Logic8/1
  Compare To Constnt9/1 -> Combinatorial Logic10/1
  Compare To Constnt10/1 -> Combinatorial Logic11/1
  Compare To Constnt11/1 -> Combinatorial Logic9/1
  Compare To Constnt12/1 -> Combinatorial Logic12/1
  Compare To Constnt13/1 -> Combinatorial Logic13/1
  Compare To Constnt14/1 -> Combinatorial Logic14/1
  Compare To Constnt15/1 -> Combinatorial Logic15/1
  Combinatorial Logic8/1 -> Logical Operator/9
  Combinatorial Logic10/1 -> Logical Operator/10
  Combinatorial Logic11/1 -> Logical Operator/11
  Combinatorial Logic9/1 -> Logical Operator/12
  Combinatorial Logic12/1 -> Logical Operator/13
  Combinatorial Logic13/1 -> Logical Operator/14
  Combinatorial Logic14/1 -> Logical Operator/15
  Combinatorial Logic15/1 -> Logical Operator/16

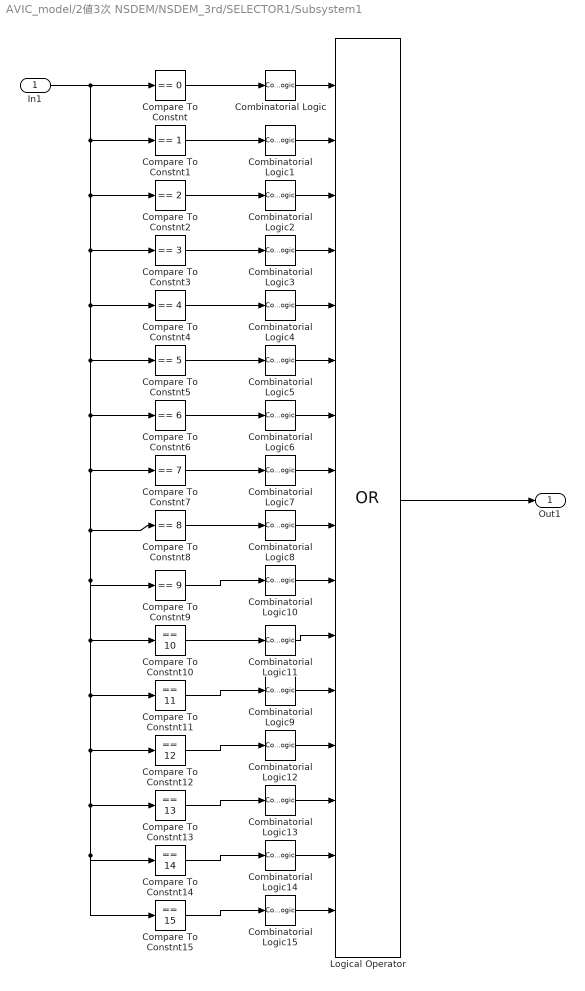
== system AVIC_model/2値3次 NSDEM/NSDEM_3rd/SELECTOR1/Subsystem1 ==
  In1 : Inport
  Combinatorial Logic : CombinatorialLogic  TruthTable=[0 0 0 0 0 0 0 0 0 0 0 0 0 0 0 0;1 0 0 0 0 0 0 0 0 0 0 0 0 0 0 0]
  Combinatorial Logic1 : CombinatorialLogic  TruthTable=[0 0 0 0 0 0 0 0 0 0 0 0 0 0 0 0; 0 1 0 0 0 0 0 0 0 0 0 0 0 0 0 0]
  Combinatorial Logic10 : CombinatorialLogic  TruthTable=[0 0 0 0 0 0 0 0 0 0 0 0 0 0 0 0;0 0 0 0 0 0 0 0 0 1 0 0 0 0 0 0]
  Combinatorial Logic11 : CombinatorialLogic  TruthTable=[0 0 0 0 0 0 0 0 0 0 0 0 0 0 0 0;0 0 0 0 0 0 0 0 0 0 1 0 0 0 0 0 ]
  Combinatorial Logic12 : CombinatorialLogic  TruthTable=[0 0 0 0 0 0 0 0 0 0 0 0 0 0 0 0;0 0 0 0 0 0 0 0 0 0 0 0 1 0 0 0]
  Combinatorial Logic13 : CombinatorialLogic  TruthTable=[0 0 0 0 0 0 0 0 0 0 0 0 0 0 0 0;0 0 0 0 0 0 0 0 0 0 0 0 0 1 0 0]
  Combinatorial Logic14 : CombinatorialLogic  TruthTable=[0 0 0 0 0 0 0 0 0 0 0 0 0 0 0 0;0 0 0 0 0 0 0 0 0 0 0 0 0 0 1 0]
  Combinatorial Logic15 : CombinatorialLogic  TruthTable=[0 0 0 0 0 0 0 0 0 0 0 0 0 0 0 0;0 0 0 0 0 0 0 0 0 0 0 0 0 0 0 1]
  Combinatorial Logic2 : CombinatorialLogic  TruthTable=[0 0 0 0 0 0 0 0 0 0 0 0 0 0 0 0;0 0 1 0 0 0 0 0 0 0 0 0 0 0 0 0]
  Combinatorial Logic3 : CombinatorialLogic  TruthTable=[0 0 0 0 0 0 0 0 0 0 0 0 0 0 0 0;0 0 0 1 0 0 0 0 0 0 0 0 0 0 0 0]
  Combinatorial Logic4 : CombinatorialLogic  TruthTable=[0 0 0 0 0 0 0 0 0 0 0 0 0 0 0 0;0 0 0 0 1 0 0 0 0 0 0 0 0 0 0 0]
  Combinatorial Logic5 : CombinatorialLogic  TruthTable=[0 0 0 0 0 0 0 0 0 0 0 0 0 0 0 0;0 0 0 0 0 1 0 0 0 0 0 0 0 0 0 0]
  Combinatorial Logic6 : CombinatorialLogic  TruthTable=[0 0 0 0 0 0 0 0 0 0 0 0 0 0 0 0;0 0 0 0 0 0 1 0 0 0 0 0 0 0 0 0]
  Combinatorial Logic7 : CombinatorialLogic  TruthTable=[0 0 0 0 0 0 0 0 0 0 0 0 0 0 0 0;0 0 0 0 0 0 0 1 0 0 0 0 0 0 0 0]
  Combinatorial Logic8 : CombinatorialLogic  TruthTable=[0 0 0 0 0 0 0 0 0 0 0 0 0 0 0 0;0 0 0 0 0 0 0 0 1 0 0 0 0 0 0 0]
  Combinatorial Logic9 : CombinatorialLogic  TruthTable=[0 0 0 0 0 0 0 0 0 0 0 0 0 0 0 0;0 0 0 0 0 0 0 0 0 0 0 1 0 0 0 0 ]
  Compare To Constnt : simulink/Logic and Bit Operations/Compare To Constant  relop===  const=0  OutDataTypeStr=boolean  ZeroCross=off
  Compare To Constnt1 : simulink/Logic and Bit Operations/Compare To Constant  relop===  const=1  OutDataTypeStr=boolean  ZeroCross=off
  Compare To Constnt10 : simulink/Logic and Bit Operations/Compare To Constant  relop===  const=10  OutDataTypeStr=boolean  ZeroCross=off
  Compare To Constnt11 : simulink/Logic and Bit Operations/Compare To Constant  relop===  const=11  OutDataTypeStr=boolean  ZeroCross=off
  Compare To Constnt12 : simulink/Logic and Bit Operations/Compare To Constant  relop===  const=12  OutDataTypeStr=boolean  ZeroCross=off
  Compare To Constnt13 : simulink/Logic and Bit Operations/Compare To Constant  relop===  const=13  OutDataTypeStr=boolean  ZeroCross=off
  Compare To Constnt14 : simulink/Logic and Bit Operations/Compare To Constant  relop===  const=14  OutDataTypeStr=boolean  ZeroCross=off
  Compare To Constnt15 : simulink/Logic and Bit Operations/Compare To Constant  relop===  const=15  OutDataTypeStr=boolean  ZeroCross=off
  Compare To Constnt2 : simulink/Logic and Bit Operations/Compare To Constant  relop===  const=2  OutDataTypeStr=boolean  ZeroCross=off
  Compare To Constnt3 : simulink/Logic and Bit Operations/Compare To Constant  relop===  const=3  OutDataTypeStr=boolean  ZeroCross=off
  Compare To Constnt4 : simulink/Logic and Bit Operations/Compare To Constant  relop===  const=4  OutDataTypeStr=boolean  ZeroCross=off
  Compare To Constnt5 : simulink/Logic and Bit Operations/Compare To Constant  relop===  const=5  OutDataTypeStr=boolean  ZeroCross=off
  Compare To Constnt6 : simulink/Logic and Bit Operations/Compare To Constant  relop===  const=6  OutDataTypeStr=boolean  ZeroCross=off
  Compare To Constnt7 : simulink/Logic and Bit Operations/Compare To Constant  relop===  const=7  OutDataTypeStr=boolean  ZeroCross=off
  Compare To Constnt8 : simulink/Logic and Bit Operations/Compare To Constant  relop===  const=8  OutDataTypeStr=boolean  ZeroCross=off
  Compare To Constnt9 : simulink/Logic and Bit Operations/Compare To Constant  relop===  const=9  OutDataTypeStr=boolean  ZeroCross=off
  Logical Operator : Logic  Operator=OR  Inputs=16  AllPortsSameDT=off  OutDataTypeStr=boolean
  Out1 : Outport
  wires:
  Logical Operator/1 -> Out1/1
  In1/1 -> Compare To Constnt/1, Compare To Constnt1/1, Compare To Constnt2/1, Compare To Constnt3/1, Compare To Constnt4/1, Compare To Constnt5/1, Compare To Constnt6/1, Compare To Constnt7/1, Compare To Constnt8/1, Compare To Constnt9/1, Compare To Constnt10/1, Compare To Constnt11/1, Compare To Constnt12/1, Compare To Constnt13/1, Compare To Constnt15/1, Compare To Constnt14/1
  Compare To Constnt/1 -> Combinatorial Logic/1
  Compare To Constnt1/1 -> Combinatorial Logic1/1
  Compare To Constnt2/1 -> Combinatorial Logic2/1
  Compare To Constnt3/1 -> Combinatorial Logic3/1
  Compare To Constnt4/1 -> Combinatorial Logic4/1
  Compare To Constnt5/1 -> Combinatorial Logic5/1
  Compare To Constnt6/1 -> Combinatorial Logic6/1
  Compare To Constnt7/1 -> Combinatorial Logic7/1
  Combinatorial Logic/1 -> Logical Operator/1
  Combinatorial Logic1/1 -> Logical Operator/2
  Combinatorial Logic2/1 -> Logical Operator/3
  Combinatorial Logic3/1 -> Logical Operator/4
  Combinatorial Logic4/1 -> Logical Operator/5
  Combinatorial Logic5/1 -> Logical Operator/6
  Combinatorial Logic6/1 -> Logical Operator/7
  Combinatorial Logic7/1 -> Logical Operator/8
  Compare To Constnt8/1 -> Combinatorial Logic8/1
  Compare To Constnt9/1 -> Combinatorial Logic10/1
  Compare To Constnt10/1 -> Combinatorial Logic11/1
  Compare To Constnt11/1 -> Combinatorial Logic9/1
  Compare To Constnt12/1 -> Combinatorial Logic12/1
  Compare To Constnt13/1 -> Combinatorial Logic13/1
  Compare To Constnt14/1 -> Combinatorial Logic14/1
  Compare To Constnt15/1 -> Combinatorial Logic15/1
  Combinatorial Logic8/1 -> Logical Operator/9
  Combinatorial Logic10/1 -> Logical Operator/10
  Combinatorial Logic11/1 -> Logical Operator/11
  Combinatorial Logic9/1 -> Logical Operator/12
  Combinatorial Logic12/1 -> Logical Operator/13
  Combinatorial Logic13/1 -> Logical Operator/14
  Combinatorial Logic14/1 -> Logical Operator/15
  Combinatorial Logic15/1 -> Logical Operator/16

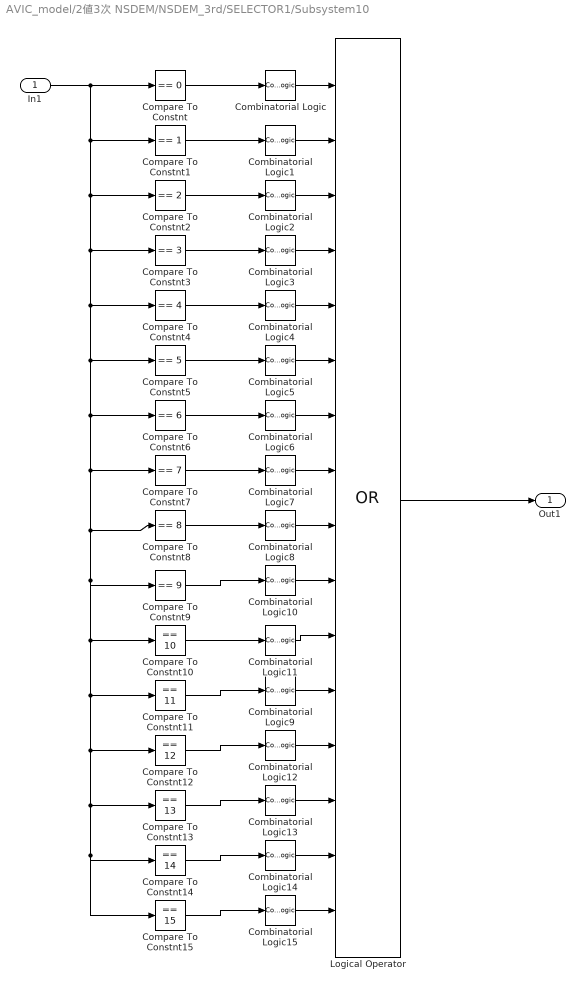
== system AVIC_model/2値3次 NSDEM/NSDEM_3rd/SELECTOR1/Subsystem10 ==
  In1 : Inport
  Combinatorial Logic : CombinatorialLogic  TruthTable=[0 0 0 0 0 0 0 0 0 0 0 0 0 0 0 0;1 0 0 0 0 0 0 0 0 0 0 0 0 0 0 0]
  Combinatorial Logic1 : CombinatorialLogic  TruthTable=[0 0 0 0 0 0 0 0 0 0 0 0 0 0 0 0; 0 1 0 0 0 0 0 0 0 0 0 0 0 0 0 0]
  Combinatorial Logic10 : CombinatorialLogic  TruthTable=[0 0 0 0 0 0 0 0 0 0 0 0 0 0 0 0;0 0 0 0 0 0 0 0 0 1 0 0 0 0 0 0]
  Combinatorial Logic11 : CombinatorialLogic  TruthTable=[0 0 0 0 0 0 0 0 0 0 0 0 0 0 0 0;0 0 0 0 0 0 0 0 0 0 1 0 0 0 0 0 ]
  Combinatorial Logic12 : CombinatorialLogic  TruthTable=[0 0 0 0 0 0 0 0 0 0 0 0 0 0 0 0;0 0 0 0 0 0 0 0 0 0 0 0 1 0 0 0]
  Combinatorial Logic13 : CombinatorialLogic  TruthTable=[0 0 0 0 0 0 0 0 0 0 0 0 0 0 0 0;0 0 0 0 0 0 0 0 0 0 0 0 0 1 0 0]
  Combinatorial Logic14 : CombinatorialLogic  TruthTable=[0 0 0 0 0 0 0 0 0 0 0 0 0 0 0 0;0 0 0 0 0 0 0 0 0 0 0 0 0 0 1 0]
  Combinatorial Logic15 : CombinatorialLogic  TruthTable=[0 0 0 0 0 0 0 0 0 0 0 0 0 0 0 0;0 0 0 0 0 0 0 0 0 0 0 0 0 0 0 1]
  Combinatorial Logic2 : CombinatorialLogic  TruthTable=[0 0 0 0 0 0 0 0 0 0 0 0 0 0 0 0;0 0 1 0 0 0 0 0 0 0 0 0 0 0 0 0]
  Combinatorial Logic3 : CombinatorialLogic  TruthTable=[0 0 0 0 0 0 0 0 0 0 0 0 0 0 0 0;0 0 0 1 0 0 0 0 0 0 0 0 0 0 0 0]
  Combinatorial Logic4 : CombinatorialLogic  TruthTable=[0 0 0 0 0 0 0 0 0 0 0 0 0 0 0 0;0 0 0 0 1 0 0 0 0 0 0 0 0 0 0 0]
  Combinatorial Logic5 : CombinatorialLogic  TruthTable=[0 0 0 0 0 0 0 0 0 0 0 0 0 0 0 0;0 0 0 0 0 1 0 0 0 0 0 0 0 0 0 0]
  Combinatorial Logic6 : CombinatorialLogic  TruthTable=[0 0 0 0 0 0 0 0 0 0 0 0 0 0 0 0;0 0 0 0 0 0 1 0 0 0 0 0 0 0 0 0]
  Combinatorial Logic7 : CombinatorialLogic  TruthTable=[0 0 0 0 0 0 0 0 0 0 0 0 0 0 0 0;0 0 0 0 0 0 0 1 0 0 0 0 0 0 0 0]
  Combinatorial Logic8 : CombinatorialLogic  TruthTable=[0 0 0 0 0 0 0 0 0 0 0 0 0 0 0 0;0 0 0 0 0 0 0 0 1 0 0 0 0 0 0 0]
  Combinatorial Logic9 : CombinatorialLogic  TruthTable=[0 0 0 0 0 0 0 0 0 0 0 0 0 0 0 0;0 0 0 0 0 0 0 0 0 0 0 1 0 0 0 0 ]
  Compare To Constnt : simulink/Logic and Bit Operations/Compare To Constant  relop===  const=0  OutDataTypeStr=boolean  ZeroCross=off
  Compare To Constnt1 : simulink/Logic and Bit Operations/Compare To Constant  relop===  const=1  OutDataTypeStr=boolean  ZeroCross=off
  Compare To Constnt10 : simulink/Logic and Bit Operations/Compare To Constant  relop===  const=10  OutDataTypeStr=boolean  ZeroCross=off
  Compare To Constnt11 : simulink/Logic and Bit Operations/Compare To Constant  relop===  const=11  OutDataTypeStr=boolean  ZeroCross=off
  Compare To Constnt12 : simulink/Logic and Bit Operations/Compare To Constant  relop===  const=12  OutDataTypeStr=boolean  ZeroCross=off
  Compare To Constnt13 : simulink/Logic and Bit Operations/Compare To Constant  relop===  const=13  OutDataTypeStr=boolean  ZeroCross=off
  Compare To Constnt14 : simulink/Logic and Bit Operations/Compare To Constant  relop===  const=14  OutDataTypeStr=boolean  ZeroCross=off
  Compare To Constnt15 : simulink/Logic and Bit Operations/Compare To Constant  relop===  const=15  OutDataTypeStr=boolean  ZeroCross=off
  Compare To Constnt2 : simulink/Logic and Bit Operations/Compare To Constant  relop===  const=2  OutDataTypeStr=boolean  ZeroCross=off
  Compare To Constnt3 : simulink/Logic and Bit Operations/Compare To Constant  relop===  const=3  OutDataTypeStr=boolean  ZeroCross=off
  Compare To Constnt4 : simulink/Logic and Bit Operations/Compare To Constant  relop===  const=4  OutDataTypeStr=boolean  ZeroCross=off
  Compare To Constnt5 : simulink/Logic and Bit Operations/Compare To Constant  relop===  const=5  OutDataTypeStr=boolean  ZeroCross=off
  Compare To Constnt6 : simulink/Logic and Bit Operations/Compare To Constant  relop===  const=6  OutDataTypeStr=boolean  ZeroCross=off
  Compare To Constnt7 : simulink/Logic and Bit Operations/Compare To Constant  relop===  const=7  OutDataTypeStr=boolean  ZeroCross=off
  Compare To Constnt8 : simulink/Logic and Bit Operations/Compare To Constant  relop===  const=8  OutDataTypeStr=boolean  ZeroCross=off
  Compare To Constnt9 : simulink/Logic and Bit Operations/Compare To Constant  relop===  const=9  OutDataTypeStr=boolean  ZeroCross=off
  Logical Operator : Logic  Operator=OR  Inputs=16  AllPortsSameDT=off  OutDataTypeStr=boolean
  Out1 : Outport
  wires:
  Logical Operator/1 -> Out1/1
  In1/1 -> Compare To Constnt/1, Compare To Constnt1/1, Compare To Constnt2/1, Compare To Constnt3/1, Compare To Constnt4/1, Compare To Constnt5/1, Compare To Constnt6/1, Compare To Constnt7/1, Compare To Constnt8/1, Compare To Constnt9/1, Compare To Constnt10/1, Compare To Constnt11/1, Compare To Constnt12/1, Compare To Constnt13/1, Compare To Constnt15/1, Compare To Constnt14/1
  Compare To Constnt/1 -> Combinatorial Logic/1
  Compare To Constnt1/1 -> Combinatorial Logic1/1
  Compare To Constnt2/1 -> Combinatorial Logic2/1
  Compare To Constnt3/1 -> Combinatorial Logic3/1
  Compare To Constnt4/1 -> Combinatorial Logic4/1
  Compare To Constnt5/1 -> Combinatorial Logic5/1
  Compare To Constnt6/1 -> Combinatorial Logic6/1
  Compare To Constnt7/1 -> Combinatorial Logic7/1
  Combinatorial Logic/1 -> Logical Operator/1
  Combinatorial Logic1/1 -> Logical Operator/2
  Combinatorial Logic2/1 -> Logical Operator/3
  Combinatorial Logic3/1 -> Logical Operator/4
  Combinatorial Logic4/1 -> Logical Operator/5
  Combinatorial Logic5/1 -> Logical Operator/6
  Combinatorial Logic6/1 -> Logical Operator/7
  Combinatorial Logic7/1 -> Logical Operator/8
  Compare To Constnt8/1 -> Combinatorial Logic8/1
  Compare To Constnt9/1 -> Combinatorial Logic10/1
  Compare To Constnt10/1 -> Combinatorial Logic11/1
  Compare To Constnt11/1 -> Combinatorial Logic9/1
  Compare To Constnt12/1 -> Combinatorial Logic12/1
  Compare To Constnt13/1 -> Combinatorial Logic13/1
  Compare To Constnt14/1 -> Combinatorial Logic14/1
  Compare To Constnt15/1 -> Combinatorial Logic15/1
  Combinatorial Logic8/1 -> Logical Operator/9
  Combinatorial Logic10/1 -> Logical Operator/10
  Combinatorial Logic11/1 -> Logical Operator/11
  Combinatorial Logic9/1 -> Logical Operator/12
  Combinatorial Logic12/1 -> Logical Operator/13
  Combinatorial Logic13/1 -> Logical Operator/14
  Combinatorial Logic14/1 -> Logical Operator/15
  Combinatorial Logic15/1 -> Logical Operator/16
